simulink model "model"  (R2021a)
settings: Solver=ode15s  StartTime=0.0  StopTime=120  RelTol=1e-3
values from neighbouring files (symbols this model uses):
  Bf = 5e-4    (= 0.0005)    [sim_model.m]
  Jt = Jm+Jl    (= 8.88e-05)    [sim_model.m]
  Ke = 0.01    [sim_model.m]
  Ra = 0.01    [sim_model.m]
undefined symbols (not defined in the file or in its folder): CQ0, CQ1, CT0, CT1, La, Td
settings Model: Creator=gpob  LastModifiedBy=gpob

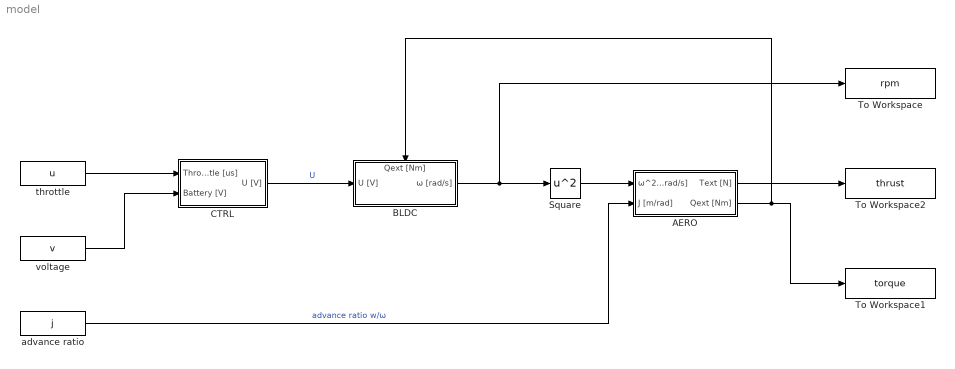
== system model ==
  AERO : Subsystem
  BLDC : Subsystem
      settings: PortSchema="{\"entries\":[{\"content\":{\"sides\":[{\"content\":{\"connectorIds\":[\"In1\"]},\"type\":\"ConnectorPlacement.EquallySpacedRectSide\",\"uuid\":\"274ecf24-0b1f-4e48-9e8c-283c14986efc\"},{\"content\":{\"connectorIds\":[\"Out1\"],\"side\":\"RIGHT\"},\"type\":\"ConnectorPlacement.EquallySpacedRectSide\",\"uuid\":\"d2296534-28d8-4f9c-a8d5-908cd34053db\"},{\"content\":{\"connectorIds\":[\"In2\"],\"side\":\"TOP\"},\"type\":\"ConnectorPlacement.EquallySpacedRectSide\",\"uuid\":\"0642ca32-8524-4238-bc0e-89fea8dfc158\"}]},\"type\":\"ConnectorPlacement.EquallySpacedConnector\",\"uuid\":\"4dc4e53c-7bd2-4fbc-a3d3-c126dfc0eebc\"}],\"packageUris\":[\"http://schema.mathworks.com/mf0/Connector/R2020b\"],\"version\":\"1.0\"}"
  CTRL : Subsystem
  Square : Math  Operator=square  SaturateOnIntegerOverflow=on
  To Workspace : ToWorkspace  VariableName=rpm  SaveFormat=Timeseries  SampleTime=-1
  To Workspace1 : ToWorkspace  VariableName=torque  SaveFormat=Timeseries  SampleTime=-1
  To Workspace2 : ToWorkspace  VariableName=thrust  SaveFormat=Timeseries  SampleTime=-1
  advance ratio : FromWorkspace  VariableName=j
  throttle : FromWorkspace  VariableName=u
  voltage : FromWorkspace  VariableName=v
  wires:
  throttle/1 -> CTRL/1(Throttle [us])
  Square/1 -> AERO/1(ω^2 [rad/s])
  voltage/1 -> CTRL/2(Battery [V])
  advance ratio/1 -> AERO/2(J [m/rad])  "advance ratio w/ω"
  AERO/2(Qext [Nm]) -> BLDC/2(Qext [Nm]), To Workspace1/1
  CTRL/1(U [V]) -> BLDC/1(U [V])  "U"
  BLDC/1(ω [rad/s]) -> To Workspace/1, Square/1
  AERO/1(Text [N]) -> To Workspace2/1

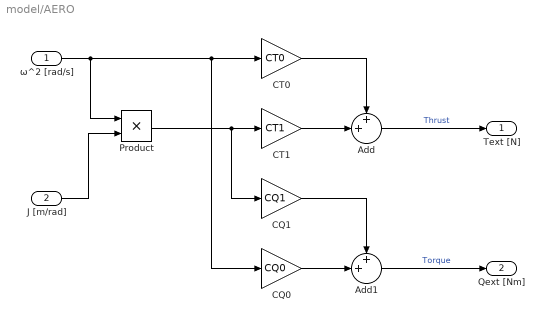
== system model/AERO ==
  ω^2 [rad/s] : Inport
  J [m/rad] : Inport  Port=2
  Add : Sum  Inputs=++|
  Add1 : Sum  Inputs=++|
  CQ0 : Gain  Gain=CQ0
  CQ1 : Gain  Gain=CQ1
  CT0 : Gain  Gain=CT0
  CT1 : Gain  Gain=CT1
  Product : Product
  Text [N] : Outport
  Qext [Nm] : Outport  Port=2
  wires:
  J [m/rad]/1 -> Product/2
  Product/1 -> CQ1/1, CT1/1
  ω^2 [rad/s]/1 -> Product/1, CQ0/1, CT0/1
  CT1/1 -> Add/2
  Add/1 -> Text [N]/1  "Thrust"
  CT0/1 -> Add/1
  Add1/1 -> Qext [Nm]/1  "Torque"
  CQ1/1 -> Add1/1
  CQ0/1 -> Add1/2

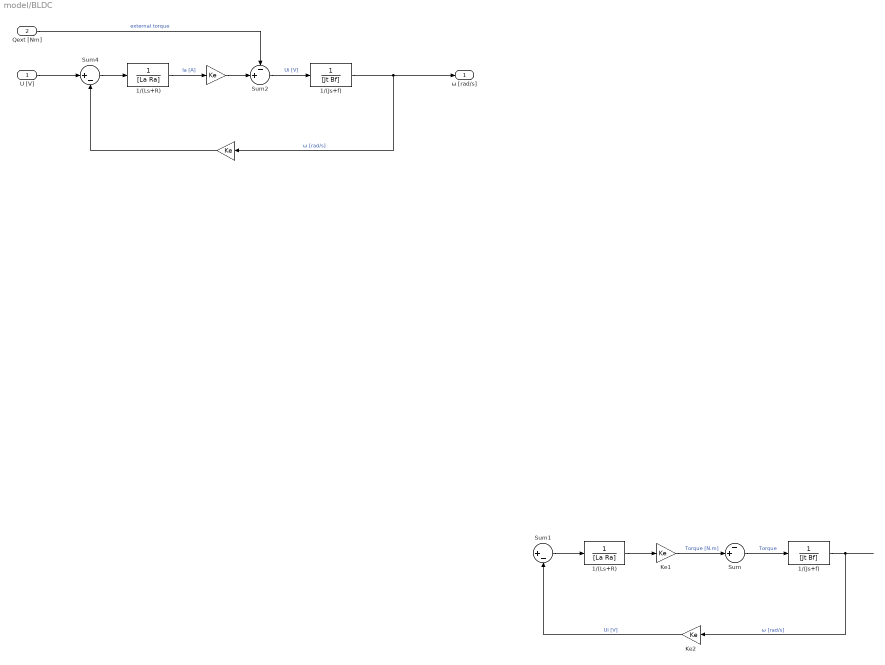
== system model/BLDC ==
  U [V] : Inport
  Qext [Nm] : Inport  Port=2
  " " : Gain  Gain=Ke
  "  " : Gain  Gain=Ke
  1/(Js+f) : TransferFcn  Denominator=[Jt Bf]
  "1/(Js+f) " : TransferFcn  Denominator=[Jt Bf]
  1/(Ls+R) : TransferFcn  Denominator=[La Ra]
  "1/(Ls+R) " : TransferFcn  Denominator=[La Ra]
  Ke1 : Gain  Gain=Ke
  Ke2 : Gain  Gain=Ke
  Sum : Sum  Inputs=-+|
  Sum1 : Sum  Inputs=|+-
  Sum2 : Sum  Inputs=-+|
  Sum4 : Sum  Inputs=|+-
  ω [rad/s] : Outport
  wires:
  Sum/1 -> 1/(Js+f)/1  "Torque"
  ? -> Sum/1  "external torque"
  1/(Js+f)/1 -> Ke2/1  "ω [rad/s]"
  Sum1/1 -> 1/(Ls+R)/1
  ? -> Sum1/1
  Ke2/1 -> Sum1/2  "Ui [V]"
  1/(Ls+R)/1 -> Ke1/1
  Ke1/1 -> Sum/2  "Torque [N.m]"
  U [V]/1 -> Sum4/1
  Sum4/1 -> "1/(Ls+R) "/1
  "1/(Ls+R) "/1 -> " "/1  "Ia [A]"
  "1/(Js+f) "/1 -> "  "/1, ω [rad/s]/1  "ω [rad/s]"
  "  "/1 -> Sum4/2
  Qext [Nm]/1 -> Sum2/1  "external torque"
  " "/1 -> Sum2/2
  Sum2/1 -> "1/(Js+f) "/1  "Ui [V]"

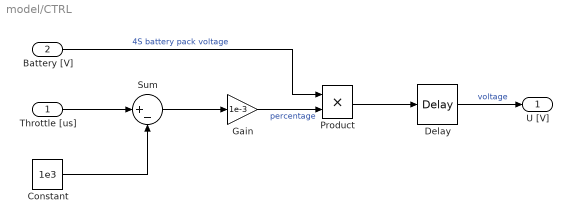
== system model/CTRL ==
  Throttle [us] : Inport
  Battery [V] : Inport  Port=2
  Constant : Constant  Value=1e3
  Delay : TransportDelay  DelayTime=Td
  Gain : Gain  Gain=1e-3
  Product : Product  Inputs=**
  Sum : Sum  Inputs=|+-
  U [V] : Outport
  wires:
  Battery [V]/1 -> Product/1  "4S battery pack voltage"
  Constant/1 -> Sum/2
  Sum/1 -> Gain/1
  Gain/1 -> Product/2  "percentage"
  Throttle [us]/1 -> Sum/1
  Product/1 -> Delay/1
  Delay/1 -> U [V]/1  "voltage"
